simulink model "IndustrialMicrogrid"  (R2023a)
settings: Solver=FixedStepDiscrete  StartTime=0.0  StopTime=10  FixedStep=Ts  RelTol=1e-3
PostLoadFcn:
  | IndustrialMicrogridInputData
  | GfmGridFormingConverterInputParameters
model workspace (MAT data in the model file):
  caseNum = 2
undefined symbols (not defined in the file): base, BESS, DiscIntNeverNeededParam, grid, Grid, gridInverter, machine, microgrid, PV, PVInverter, PVTransformer, scrFactorRg, scrFactorXg, transformer, Ts
libraries: ee_lib x112, eeGeneralControl x104, nesl_utility_internal x64, simulink x56, nesl_utility x37, fl_lib x29, slpidlib x13, eeTransforms x11, eeTotalHarmonicDistorsion x8, eeRmsMeasurement x4, eeSinusoidalMeasurement x4, simulink_extras x2
(part 1 of 14)
CloseFcn:
  | figure1 = findobj('Type', 'figure', 'Name','h1_IndustrialMicrogrid');
  | figure2 = findobj('Type', 'figure', 'Name','h2_IndustrialMicrogrid');
  | figure3 = findobj('Type', 'figure', 'Name','h3_IndustrialMicrogrid');
  | figure4 = findobj('Type', 'figure', 'Name','h4_IndustrialMicrogrid');
  | figure5 = findobj('Type', 'figure', 'Name','h5_IndustrialMicrogrid');
  | close(figure1);
  | close(figure2);
  | close(figure3);
  | close(figure4);
  | close(figure5);
  | clear figure1 figure2 figure3 figure4 figure5
  | clear BESS closedLoop controller currentLoopPole
  | clear fsw_V geometricMean grid Grid inverter KI_PVPLL
  | clear KP_PVPLL logsout_ee_microgrid_resynchronization
  | clear Microgrid PrimaryreactancePV PrimaryresistancePV
  | clear remainingPowerPerString SecondaryreactancePV
  | clear SecondaryresistancePV sensor simlog_ee_microgrid_resynchronization
  | clear simulation solarPanel solarPlant TransformerPrimaryVoltagePV
  | clear TransformerRatingPV TransformerSecondaryVoltagePV
  | clear Ts Ts_V Solar logsout_ee_microgrid_for_mines simlog_ee_microgrid_for_mines
  | clear ans AuxiliaryLoad base BESSCost1 BESSCost2 BESSCost3
  | clear BESSCost4 BESSKVAs1 BESSKVAs2 BESSKVAs3 BESSKVAs4
  | clear BESSMVA1 BESSMVA2 caseNum Conveyor Diesel_cost_s1
  | clear Diesel_cost_s1_yr Diesel_cost_s2 Diesel_cost_s2_yr
  | clear Diesel_cost_s3 Diesel_cost_s3_yr Diesel_cost_s4
  | clear Diesel_cost_s4_yr diesel_litre_USD Diesel_loading_100percent
  | clear Diesel_loading_25percent Diesel_loading_50percent Diesel_loading_75percent
  | clear Diesel_s1 Diesel_s2 Diesel_s3 Diesel_s4 DieselCost1 DieselCost2 DieselCost3
  | clear DieselCost4 DieselKVAs1 DieselKVAs2 DieselKVAs3 DieselKVAs4 DieselMVA
  | clear disturbanceTime DrillingLoad1 DrillingLoad2a DrillingLoad2b Grid1Limited Grid1MVA
  | clear Grid2Limited gridInverter h11a_IndustrialMicrogrid h22a_IndustrialMicrogrid
  | clear h2a_IndustrialMicrogrid imaginaryPart LightingLoad localSolverSampleTime logsout1
  | clear logsout2 logsout3 logsout4 logsout5 logsout_activeloss1 logsout_activeloss2
  | clear logsout_activeloss3 logsout_activeloss4 logsout_activeloss5 logsout_freqmax1
  | clear logsout_freqmax2 logsout_freqmax3 logsout_freqmax4 logsout_freqmax5 logsout_freqmin1
  | clear logsout_freqmin2 logsout_freqmin3 logsout_freqmin4 logsout_freqmin5 logsout_IndustrialMicrogrid
  | clear logsout_LoadTHD1 logsout_LoadTHD2 logsout_LoadTHD3 logsout_LoadTHD4 logsout_LoadTHD5
  | clear logsout_MaxLoadVoltage1 logsout_MaxLoadVoltage2 logsout_MaxLoadVoltage3 logsout_MaxLoadVoltage4
  | clear logsout_MaxLoadVoltage5 logsout_MinLoadVoltage1 logsout_MinLoadVoltage2 logsout_MinLoadVoltage3
  | clear logsout_MinLoadVoltage4 logsout_MinLoadVoltage5 logsout_PCCTHD1 logsout_PCCTHD2
  | clear logsout_PCCTHD3 logsout_PCCTHD4 logsout_PCCTHD5 logsout_reactiveloss1
  | clear logsout_reactiveloss2 logsout_reactiveloss3 logsout_reactiveloss4 logsout_reactiveloss5
  | clear logsout_volmax1 logsout_volmax2 logsout_volmax3 logsout_volmax4 logsout_volmax5
  | clear logsout_volmin1 logsout_volmin2 logsout_volmin3 logsout_volmin4 logsout_volmin5
  | clear machine Machine Micorgrid microgrid op opCase5 ProcessingMotorLoad PV PVCost1
  | clear PVCost2 PVCost3 PVCost4 PVInverter PVKVAs1 PVKVAs2 PVKVAs3 PVKVAs4 PVMVA
  | clear PVTransformer realPart scrFactorRg scrFactorXg scrOut shortCircuit
  | clear simlog_IndustrialMicrogrid simulationTime Solar_cell systemSCR T_on testCondition
  | clear TotalCost1 TotalCost2 TotalCost3 TotalCost4 TotalMG1Load TotalMG2Generation
  | clear TotalMG2Load transformer TransmissionLine tStart tStop voltageLimit voltageLimitMax
  | clear voltageLimitMin XbyROut XbyRtempFactor xlim xticks
  | clear grid Grid gridInverter machine microgrid Microgrid microgridSubsystems PV PVTransformer resultsSubsystems signalRoomSubsystems Ts topLevelSubsystems transformer opCtrlRoomSubsystems
  | clear opCase1 opCase2 opCase3 opCase4 opCase5
Description:
  | Industrial  Microgrid
settings Model: PauseTimes=1  Creator=The MathWorks, Inc.  LastModifiedBy=greed
settings SolverCC: AlgebraicLoopSolver=TrustRegion
settings DataIOCC: ExternalInput=getinputstruct(op)  InitialState=getstatestruct(op)  LoadExternalInput=on  LoadInitialState=on  SaveOutput=off  SaveTime=off  SignalLoggingName=logsout_IndustrialMicrogrid  OutputTimes=[0:1.1*3*Voc/(1*2000):1.1*3*Voc/1]  ReturnWorkspaceOutputsName=simoutData
settings OptimizationCC: ReuseModelBlockBuffer=off
settings DebuggingCC: UnconnectedInputMsg=warning  UnconnectedOutputMsg=warning  UnconnectedLineMsg=warning  StateNameClashWarn=warning  SubsystemReferenceDiagnosticForUnitTest=warning  ArithmeticOperatorsInVariantConditions=warning
settings HardwareCC: ProdBitPerPointer=32  ProdBitPerSizeT=32  ProdBitPerPtrDiffT=32  ProdWordSize=32  ProdHWDeviceType=Intel->x86-32 (Windows32)
settings ModelReferenceCC: EnableRefExpFcnMdlSchedulingChecks=on  PropagateSignalLabelsOutOfModel=off
settings SFSimCC: CustomCodeUndefinedFunction=UseInterfaceOnly
settings RTWCC: DLArmComputeVersion=19.05
settings CodeAppCC: StateflowObjectComments=on
settings SimscapeCC: SimscapeNominalValues="[{\"value\":\"1\",\"unit\":\"A\"},{\"value\":\"1\",\"unit\":\"bar\"},{\"value\":\"1\",\"unit\":\"cm^2\"},{\"value\":\"1\",\"unit\":\"cm^3/s\"},{\"value\":\"1\",\"unit\":\"kJ/kg\"},{\"value\":\"1\",\"unit\":\"kW\"},{\"value\":\"1\",\"unit\":\"l\"},{\"value\":\"1\",\"unit\":\"N\"},{\"value\":\"1\",\"unit\":\"N*m\"},{\"value\":\"1e3\",\"unit\":\"V\"}]"  SimscapeLogType=all  SimscapeLogSimulationStatistics=on  SimscapeLogName=simlog_IndustrialMicrogrid  SimscapeLogLimitData=off

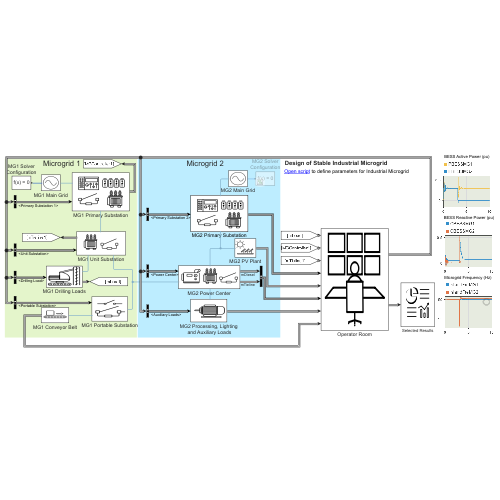
[thumbnail: Simulink's stored preview of the top-level diagram]
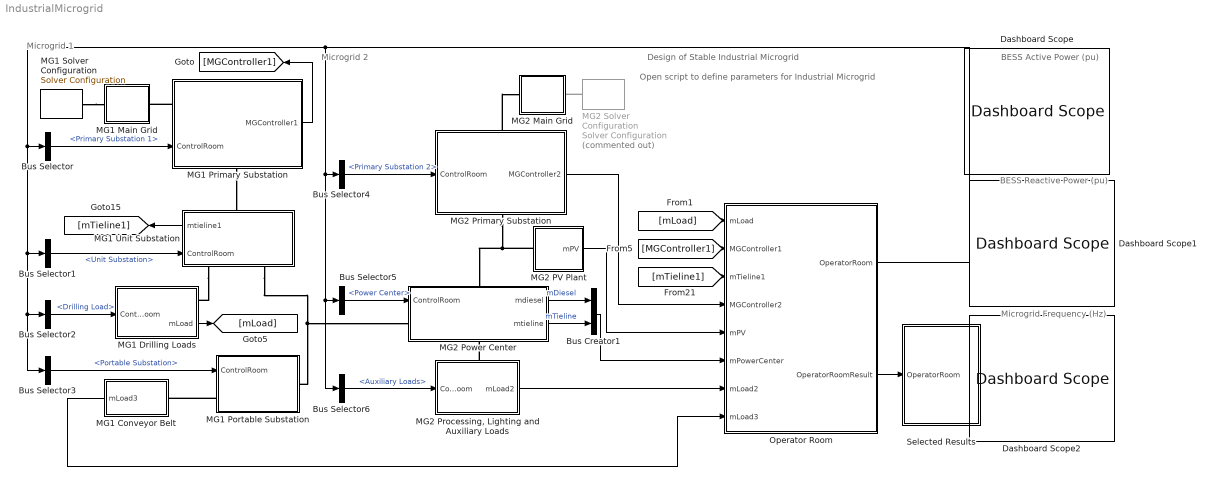
== system IndustrialMicrogrid ==
  note: BESS Active Power (pu)
  note: Microgrid 1
  note: Microgrid 2
  note: Design of Stable Industrial Microgrid
  note: Open script to define parameters for Industrial Microgrid
  note: BESS Reactive Power (pu)
  note: Microgrid Frequency (Hz)
  Bus Creator1 : BusCreator  Inputs=2
  Bus Selector : BusSelector  OutputSignals=Primary Substation 1
  Bus Selector1 : BusSelector  OutputSignals=Unit Substation
  Bus Selector2 : BusSelector  OutputSignals=Drilling Load
  Bus Selector3 : BusSelector  OutputSignals=Portable Substation
  Bus Selector4 : BusSelector  OutputSignals=Primary Substation 2
  Bus Selector5 : BusSelector  OutputSignals=Power Center
  Bus Selector6 : BusSelector  OutputSignals=Auxiliary Loads
  Dashboard Scope : DashboardScope
  Dashboard Scope1 : DashboardScope
  Dashboard Scope2 : DashboardScope
  MG1 Conveyor Belt : Subsystem
      mask Display: image('$imagefile'); % Use "Edit Image" on toolstrip to change.
  MG1 Drilling Loads : Subsystem
      settings: PortSchema="{\"entries\":[{\"content\":{\"sides\":[{\"content\":{\"connectorIds\":[\"In1\"]},\"type\":\"ConnectorPlacement.EquallySpacedRectSide\",\"uuid\":\"8bde343d-193d-4d8c-8111-593ba83965eb\"},{\"content\":{\"connectorIds\":[\"RConn1\",\"Out1\"],\"side\":\"RIGHT\"},\"type\":\"ConnectorPlacement.EquallySpacedRectSide\",\"uuid\":\"2ced8eac-92b1-40fd-b9a3-0c7198a29bec\"},{\"content\":{\"connectorIds\":[],\"side\":\"TOP\"},\"type\":\"ConnectorPlacement.EquallySpacedRectSide\",\"uuid\":\"35b22a7d-ddf4-481a-bb03-3d287fb8e47a\"}]},\"type\":\"ConnectorPlacement.EquallySpacedConnector\",\"uuid\":\"38972ecb-e14c-4d7a-b334-c84224067a82\"}],\"packageUris\":[\"http://schema.mathworks.com/mf0/Connector/R2020b\"],\"version\":\"1.0\"}"
      mask Display: image('$imagefile'); % Use "Edit Image" on toolstrip to change.
  MG1 Main Grid : Subsystem
      mask Display: image('$imagefile'); % Use "Edit Image" on toolstrip to change.
  MG1 Portable Substation : Subsystem
      mask Display: image('$imagefile'); % Use "Edit Image" on toolstrip to change.
  MG1 Primary Substation : Subsystem
      settings: PortSchema="{\"entries\":[{\"content\":{\"sides\":[{\"content\":{\"connectorIds\":[\"LConn1\",\"In1\"]},\"type\":\"ConnectorPlacement.EquallySpacedRectSide\",\"uuid\":\"62c365b4-4668-43f4-b939-0cfa584e512e\"},{\"content\":{\"connectorIds\":[\"Out1\"],\"side\":\"RIGHT\"},\"type\":\"ConnectorPlacement.EquallySpacedRectSide\",\"uuid\":\"025ab869-e565-436b-82b8-3d49f2a71b4a\"},{\"content\":{\"side\":\"TOP\"},\"type\":\"ConnectorPlacement.EquallySpacedRectSide\",\"uuid\":\"be91cdb0-9ff1-46ba-9800-55b3072c8f0d\"},{\"content\":{\"connectorIds\":[\"RConn1\"],\"side\":\"BOTTOM\"},\"type\":\"ConnectorPlacement.EquallySpacedRectSide\",\"uuid\":\"d77b7477-2bba-487e-be1b-8a281c49c410\"}]},\"type\":\"ConnectorPlacement.EquallySpacedConnector\",\"uuid\":\"adc0c184-ac84-487f-a22d-12a7e7737206\"}],\"packageUris\":[\"http://schema.mathworks.com/mf0/Connector/R2020b\"],\"version\":\"1.0\"}"
      mask Display: image('$imagefile'); % Use "Edit Image" on toolstrip to change.
  MG1 Solver Configuration : nesl_utility_internal/Solver Configuration  PhysicalDomain=network_engine_domain  SubClassName=solver  LeftPortType=input  RightPortType=generic  Tones=[]  Harmonics=[]  SimulateNoise=off  Profile=off  UseLocalSampling=off  EnableSwitchedLinearOptims=on  FrequencyDomain=off  UseCCode=off  RelTol=0.001  AbsTol=1e-06  MinStep=1e-09  ToWorkspace=off  RevertToSquareIcSolve=off  NumHomotopyIterations=100  PhasorMode=off  PhasorModeNumHarmonics=1  ConsistencySolver=NEWTON_FTOL  IndexReductionMethod=None  DoDC=off  ResidualTolerance=1e-07  ConsistencyTolSource=GLOBAL  ConsistencyAbsTol=0.001  ConsistencyRelTol=0.001  ConsistencyTolFactor=0.001  UseLocalSolver=on  LocalSolverChoice=NE_PARTITIONING_ADVANCER  ResolveIndetEquations=on  FunctionEvalNumThread=1  LocalSolverSampleTime=Ts  DoFixedCost=on  MaxNonlinIter=3  MaxModeIter=2  ComputeImpulses=off  ImpulseIterations=1  LinearAlgebra=auto  LinearAlgebraNumThread=0  EquationFormulation=NE_TIME_EF  DelaysMemoryBudget=1024  AutomaticFiltering=off  FilteringTimeConstant=0.001  PartitionStorageMethod=EXHAUSTIVE  PartitionMemoryBudget=1024  PartitionMethod=ROBUST
  MG1 Unit Substation : Subsystem
      settings: PortSchema="{\"entries\":[{\"content\":{\"sides\":[{\"content\":{\"connectorIds\":[\"Out1\",\"In1\"]},\"type\":\"ConnectorPlacement.EquallySpacedRectSide\",\"uuid\":\"75ac93d6-cc6a-445c-be45-fffab924bfd7\"},{\"content\":{\"side\":\"RIGHT\"},\"type\":\"ConnectorPlacement.EquallySpacedRectSide\",\"uuid\":\"e5c53324-ad77-49da-90c4-df6ba5240965\"},{\"content\":{\"connectorIds\":[\"LConn1\"],\"side\":\"TOP\"},\"type\":\"ConnectorPlacement.EquallySpacedRectSide\",\"uuid\":\"55d13e88-751b-43c7-af74-511b72769f16\"},{\"content\":{\"connectorIds\":[\"RConn1\",\"RConn2\"],\"side\":\"BOTTOM\"},\"type\":\"ConnectorPlacement.EquallySpacedRectSide\",\"uuid\":\"b5dd3cb9-7b98-4c05-8dd8-d8e7dc6e0ca9\"}]},\"type\":\"ConnectorPlacement.EquallySpacedConnector\",\"uuid\":\"f5372cf6-2eab-4920-89a5-bce690804323\"}],\"packageUris\":[\"http://schema.mathworks.com/mf0/Connector/R2020b\"],\"version\":\"1.0\"}"
      mask Display: image('$imagefile'); % Use "Edit Image" on toolstrip to change.
  MG2 Main Grid : Subsystem
      mask Display: image('$imagefile'); % Use "Edit Image" on toolstrip to change.
  MG2 PV Plant : Subsystem
      mask Display: image('$imagefile'); % Use "Edit Image" on toolstrip to change.
  MG2 Power Center : Subsystem
      settings: PortSchema="{\"entries\":[{\"content\":{\"sides\":[{\"content\":{\"connectorIds\":[\"In1\",\"LConn1\"]},\"type\":\"ConnectorPlacement.EquallySpacedRectSide\",\"uuid\":\"75ac93d6-cc6a-445c-be45-fffab924bfd7\"},{\"content\":{\"connectorIds\":[\"Out1\",\"Out2\"],\"side\":\"RIGHT\"},\"type\":\"ConnectorPlacement.EquallySpacedRectSide\",\"uuid\":\"e5c53324-ad77-49da-90c4-df6ba5240965\"},{\"content\":{\"connectorIds\":[\"LConn2\"],\"side\":\"TOP\"},\"type\":\"ConnectorPlacement.EquallySpacedRectSide\",\"uuid\":\"55d13e88-751b-43c7-af74-511b72769f16\"},{\"content\":{\"connectorIds\":[\"RConn1\"],\"side\":\"BOTTOM\"},\"type\":\"ConnectorPlacement.EquallySpacedRectSide\",\"uuid\":\"640896eb-fba6-44de-a484-c435c51ba156\"}]},\"type\":\"ConnectorPlacement.EquallySpacedConnector\",\"uuid\":\"f5372cf6-2eab-4920-89a5-bce690804323\"}],\"packageUris\":[\"http://schema.mathworks.com/mf0/Connector/R2020b\"],\"version\":\"1.0\"}"
      mask Display: image('$imagefile'); % Use "Edit Image" on toolstrip to change.
  MG2 Primary Substation : Subsystem
      settings: PortSchema="{\"entries\":[{\"content\":{\"sides\":[{\"content\":{\"connectorIds\":[\"In1\"]},\"type\":\"ConnectorPlacement.EquallySpacedRectSide\",\"uuid\":\"a418e4cb-bf63-409d-8e7f-8f8f381466aa\"},{\"content\":{\"connectorIds\":[\"Out1\"],\"side\":\"RIGHT\"},\"type\":\"ConnectorPlacement.EquallySpacedRectSide\",\"uuid\":\"36367aff-fc5a-4e64-9409-cab392a29391\"},{\"content\":{\"connectorIds\":[\"LConn1\"],\"side\":\"TOP\"},\"type\":\"ConnectorPlacement.EquallySpacedRectSide\",\"uuid\":\"594bd116-4459-44f1-a349-157ea2209965\"},{\"content\":{\"connectorIds\":[\"RConn1\"],\"side\":\"BOTTOM\"},\"type\":\"ConnectorPlacement.EquallySpacedRectSide\",\"uuid\":\"1ed5e2c8-52ef-46e8-a3fd-2e92dd02a56f\"}]},\"type\":\"ConnectorPlacement.EquallySpacedConnector\",\"uuid\":\"f6551318-b622-4306-bcf5-d56dd1a3ddaf\"}],\"packageUris\":[\"http://schema.mathworks.com/mf0/Connector/R2020b\"],\"version\":\"1.0\"}"
      mask Display: image('$imagefile'); % Use "Edit Image" on toolstrip to change.
  "MG2 Processing, Lighting and Auxiliary Loads" : Subsystem
      settings: PortSchema="{\"entries\":[{\"content\":{\"sides\":[{\"content\":{\"connectorIds\":[\"In1\"]},\"type\":\"ConnectorPlacement.EquallySpacedRectSide\",\"uuid\":\"8bde343d-193d-4d8c-8111-593ba83965eb\"},{\"content\":{\"connectorIds\":[\"Out1\"],\"side\":\"RIGHT\"},\"type\":\"ConnectorPlacement.EquallySpacedRectSide\",\"uuid\":\"2ced8eac-92b1-40fd-b9a3-0c7198a29bec\"},{\"content\":{\"connectorIds\":[\"LConn1\"],\"side\":\"TOP\"},\"type\":\"ConnectorPlacement.EquallySpacedRectSide\",\"uuid\":\"35b22a7d-ddf4-481a-bb03-3d287fb8e47a\"}]},\"type\":\"ConnectorPlacement.EquallySpacedConnector\",\"uuid\":\"38972ecb-e14c-4d7a-b334-c84224067a82\"}],\"packageUris\":[\"http://schema.mathworks.com/mf0/Connector/R2020b\"],\"version\":\"1.0\"}"
      mask Display: image('$imagefile'); % Use "Edit Image" on toolstrip to change.
  MG2 Solver Configuration : nesl_utility_internal/Solver Configuration  Commented=on  PhysicalDomain=network_engine_domain  SubClassName=solver  LeftPortType=input  RightPortType=generic  Tones=[]  Harmonics=[]  SimulateNoise=off  Profile=off  UseLocalSampling=off  EnableSwitchedLinearOptims=on  FrequencyDomain=off  UseCCode=off  RelTol=0.001  AbsTol=1e-06  MinStep=1e-09  ToWorkspace=off  RevertToSquareIcSolve=off  NumHomotopyIterations=100  PhasorMode=off  PhasorModeNumHarmonics=1  ConsistencySolver=NEWTON_FTOL  IndexReductionMethod=None  DoDC=off  ResidualTolerance=1e-07  ConsistencyTolSource=GLOBAL  ConsistencyAbsTol=0.001  ConsistencyRelTol=0.001  ConsistencyTolFactor=0.001  UseLocalSolver=on  LocalSolverChoice=NE_PARTITIONING_ADVANCER  ResolveIndetEquations=on  FunctionEvalNumThread=1  LocalSolverSampleTime=Ts  DoFixedCost=on  MaxNonlinIter=3  MaxModeIter=2  ComputeImpulses=off  ImpulseIterations=1  LinearAlgebra=auto  LinearAlgebraNumThread=0  EquationFormulation=NE_TIME_EF  DelaysMemoryBudget=1024  AutomaticFiltering=off  FilteringTimeConstant=0.001  PartitionStorageMethod=EXHAUSTIVE  PartitionMemoryBudget=1024  PartitionMethod=ROBUST
  Operator Room : Subsystem
      mask Display: image('$imagefile'); % Use "Edit Image" on toolstrip to change.
  Selected Results : Subsystem
      mask Display: image('$imagefile'); % Use "Edit Image" on toolstrip to change.
  wires:
  MG1 Primary Substation/1(MGController1) -> [MGController1]
  MG1 Drilling Loads/1(mLoad) -> [mLoad]
  Bus Selector1/1 -> MG1 Unit Substation/1(ControlRoom)  "<Unit Substation>"
  Bus Selector2/1 -> MG1 Drilling Loads/1(ControlRoom)  "<Drilling Load>"
  Bus Selector3/1 -> MG1 Portable Substation/1(ControlRoom)  "<Portable Substation>"
  [mLoad] -> Operator Room/1(mLoad)
  "MG2 Processing, Lighting and Auxiliary Loads"/1(mLoad2) -> Operator Room/7(mLoad2)
  MG2 Primary Substation/1(MGController2) -> Operator Room/4(MGController2)
  MG2 PV Plant/1(mPV) -> Operator Room/5(mPV)
  [MGController1] -> Operator Room/2(MGController1)
  MG1 Conveyor Belt/1(mLoad3) -> Operator Room/8(mLoad3)
  MG1 Unit Substation/1(mtieline1) -> [mTieline1]
  Operator Room/1(OperatorRoom) -> Bus Selector6/1, Bus Selector5/1, Bus Selector4/1, Bus Selector2/1, Bus Selector3/1, Bus Selector1/1, Bus Selector/1
  Bus Selector5/1 -> MG2 Power Center/1(ControlRoom)  "<Power Center>"
  Bus Selector6/1 -> "MG2 Processing, Lighting and Auxiliary Loads"/1(ControlRoom)  "<Auxiliary Loads>"
  Bus Selector/1 -> MG1 Primary Substation/1(ControlRoom)  "<Primary Substation 1>"
  MG2 Power Center/1(mdiesel) -> Bus Creator1/1  "mDiesel"
  MG2 Power Center/2(mtieline) -> Bus Creator1/2  "mTieline"
  Operator Room/2(OperatorRoomResult) -> Selected Results/1(OperatorRoom)
  [mTieline1] -> Operator Room/3(mTieline1)
  Bus Creator1/1 -> Operator Room/6(mPowerCenter)
  Bus Selector4/1 -> MG2 Primary Substation/1(ControlRoom)  "<Primary Substation 2>"
  connections:
  MG1 Primary Substation/LConn1 -- MG1 Main Grid/RConn1
  MG1 Solver Configuration/RConn1 -- MG1 Main Grid/LConn1
  MG1 Primary Substation/RConn1 -- MG1 Unit Substation/LConn1
  MG2 Solver Configuration/RConn1 -- MG2 Main Grid/LConn1
  "MG2 Processing, Lighting and Auxiliary Loads"/LConn1 -- MG2 Power Center/RConn1
  MG2 Primary Substation/LConn1 -- MG2 Main Grid/RConn1
  MG1 Unit Substation/RConn1 -- MG1 Drilling Loads/RConn1
  MG1 Unit Substation/RConn2 -- MG1 Portable Substation/RConn1 -- MG2 Power Center/LConn1
  MG1 Portable Substation/LConn1 -- MG1 Conveyor Belt/LConn1
  MG2 Primary Substation/RConn1 -- MG2 PV Plant/LConn1 -- MG2 Power Center/LConn2

== system IndustrialMicrogrid/MG1 Conveyor Belt ==
  Average-Value Rectifier (Three-Phase) : ee_lib/Semiconductors & Converters/Converters/Average-Value Rectifier (Three-Phase)  port_option=ee.enum.threePhasePort.composite  frequency_option=ee.enum.converters.frequency.variable  VRated=microgrid.powerCenterTransformerSecondaryVoltage V  FRated=60 Hz  Pfixed=5e3 W
      settings: InternalSimscapePortConfiguration="{\"Bottom\":[],\"Left\":[{\"id\":\"N\",\"label\":\"~\",\"type\":\"foundation.electrical.three_phase\"}],\"Right\":[{\"id\":\"p\",\"label\":\"+\",\"type\":\"foundation.electrical.electrical\"},{\"id\":\"n\",\"label\":\"-\",\"type\":\"foundation.electrical.electrical\"}],\"Top\":[]}"
  Low-Pass Filter (Discrete or Continuous)1 : eeGeneralControl/Low-Pass Filter (Discrete or Continuous)  K=1  T=0.02  B=inf  A=-inf  init_option=Inherited from block input  x0=0  Ts=Ts
  Low-Pass Filter (Discrete or Continuous)2 : eeGeneralControl/Low-Pass Filter (Discrete or Continuous)  K=1  T=0.02  B=inf  A=-inf  init_option=Inherited from block input  x0=0  Ts=Ts
  PS-Simulink Converter6 : nesl_utility_internal/PS-Simulink Converter  PhysicalDomain=network_engine_domain  SubClassName=ps_output  LeftPortType=input  RightPortType=output  PseudoPeriodic=off  Frequencies=[]  VectorFormat=1-D array  Unit=MW  AffineConversion=off
  PS-Simulink Converter7 : nesl_utility_internal/PS-Simulink Converter  PhysicalDomain=network_engine_domain  SubClassName=ps_output  LeftPortType=input  RightPortType=output  PseudoPeriodic=off  Frequencies=[]  VectorFormat=1-D array  Unit=MV*A  AffineConversion=off
  Power Sensor (Three-Phase)1 : ee_lib/Sensors & Transducers/Power Sensor (Three-Phase)  load_type=ee.enum.passive.type_balanced.balanced  f0=60 Hz  config=ee.enum.with_neutral.no  rho=1
      settings: InternalSimscapePortConfiguration="{\"Bottom\":[],\"Left\":[{\"id\":\"N1\",\"label\":\"~1\",\"type\":\"foundation.electrical.three_phase\"}],\"Right\":[{\"id\":\"N2\",\"label\":\"~2\",\"type\":\"foundation.electrical.three_phase\"}],\"Top\":[{\"id\":\"Pm\",\"label\":\"P\",\"type\":\"output\"},{\"id\":\"Qm\",\"label\":\"Q\",\"type\":\"output\"}]}"
  Resistor : ee_lib/Passive/Resistor  R=2500 Ohm  enable_R_tol=0  R_tol=5  tol_distribution=1  nSigma=4  enable_operating_limits=0  operating_limit_action=2  power_rating=1 W  max_working_voltage=100 V  enable_faults=ee.enum.enable.no  fault_action=simscape.enum.assert.action.none  R_faulted=inf Ohm  fault_trigger=ee.enum.faults.faultTrigger.temporal  t_fault=1 s  max_permissible_current=1 A  t_fail_on_current=1 s  noise_mode=0  Tdevice=25 degC  sample_time=1e-3 s  repeatability=1  user_seed=0  auto_seed=3499211588  power_derating_T1=70 degC  power_derating_T2=155 degC  operating_temperature_range_vec=[-50, 150] degC  alpha=3.93e-3 1/K  Tmeas=25 degC  thermal_mass=100 J/K  temperature_specify=off  temperature_priority=High  temperature=298.15 K  temperature_nominal_specify=off  temperature_nominal_unit=K  temperature_nominal_value=1
  ~ : PMIOPort  Side=Left
  Out Bus Element2 : Outport  PortName=mLoad3  Element=activepower
  Out Bus Element3 : Outport  PortName=mLoad3  Element=reactivepower
  wires:
  PS-Simulink Converter6/1 -> Low-Pass Filter (Discrete or Continuous)1/1
  PS-Simulink Converter7/1 -> Low-Pass Filter (Discrete or Continuous)2/1
  Low-Pass Filter (Discrete or Continuous)1/1 -> Out Bus Element2/1
  Low-Pass Filter (Discrete or Continuous)2/1 -> Out Bus Element3/1
  connections:
  Resistor/LConn1 -- Average-Value Rectifier (Three-Phase)/RConn1
  Resistor/RConn1 -- Average-Value Rectifier (Three-Phase)/RConn2
  ~/RConn1 -- Power Sensor (Three-Phase)1/LConn1
  Power Sensor (Three-Phase)1/RConn1 -- Average-Value Rectifier (Three-Phase)/LConn1
  Power Sensor (Three-Phase)1/LConn2 -- PS-Simulink Converter6/LConn1
  Power Sensor (Three-Phase)1/LConn3 -- PS-Simulink Converter7/LConn1

== system IndustrialMicrogrid/MG1 Drilling Loads ==
  Bus Element In3 : Inport  PortName=ControlRoom  Element=Load2aControl
  Bus Element In1 : Inport  PortName=ControlRoom  Element=Load1Control
  Bus Element In2 : Inport  PortName=ControlRoom  Element=Load2bControl
  Circuit Breaker (Three-Phase)1 : ee_lib/Switches & Breakers/Circuit Breaker (Three-Phase)  R_closed=0.001 Ohm  G_open=1e-6 1/Ohm  threshold=0.5 V  breaker_behavior=ee.enum.switches.breakerBehavior.zeroCrossingEnable
      settings: InternalSimscapePortConfiguration="{\"Bottom\":[],\"Left\":[{\"id\":\"vT\",\"label\":\"vT\",\"type\":\"input\"},{\"id\":\"N1\",\"label\":\"~1\",\"type\":\"foundation.electrical.three_phase\"}],\"Right\":[{\"id\":\"N2\",\"label\":\"~2\",\"type\":\"foundation.electrical.three_phase\"}],\"Top\":[]}"
  Circuit Breaker (Three-Phase)2 : ee_lib/Switches & Breakers/Circuit Breaker (Three-Phase)  R_closed=0.001 Ohm  G_open=1e-6 1/Ohm  threshold=0.5 V  breaker_behavior=ee.enum.switches.breakerBehavior.zeroCrossingEnable
      settings: InternalSimscapePortConfiguration="{\"Bottom\":[],\"Left\":[{\"id\":\"vT\",\"label\":\"vT\",\"type\":\"input\"},{\"id\":\"N1\",\"label\":\"~1\",\"type\":\"foundation.electrical.three_phase\"}],\"Right\":[{\"id\":\"N2\",\"label\":\"~2\",\"type\":\"foundation.electrical.three_phase\"}],\"Top\":[]}"
  Circuit Breaker (Three-Phase)3 : ee_lib/Switches & Breakers/Circuit Breaker (Three-Phase)  R_closed=0.001 Ohm  G_open=1e-6 1/Ohm  threshold=0.5 V  breaker_behavior=ee.enum.switches.breakerBehavior.zeroCrossingEnable
      settings: InternalSimscapePortConfiguration="{\"Bottom\":[],\"Left\":[{\"id\":\"vT\",\"label\":\"vT\",\"type\":\"input\"},{\"id\":\"N1\",\"label\":\"~1\",\"type\":\"foundation.electrical.three_phase\"}],\"Right\":[{\"id\":\"N2\",\"label\":\"~2\",\"type\":\"foundation.electrical.three_phase\"}],\"Top\":[]}"
  Electrical Reference1 : fl_lib/Electrical/Electrical Elements/Electrical Reference
  Electrical Reference2 : fl_lib/Electrical/Electrical Elements/Electrical Reference
  Load Measurements1 : Subsystem
  Simulink-PS Converter1 : nesl_utility_internal/Simulink-PS Converter  PhysicalDomain=network_engine_domain  SubClassName=ps_input  LeftPortType=input  RightPortType=output  PseudoPeriodic=off  Frequencies=[]  NoiseDistribution=none  NoiseParameters=[]  Unit=1  AffineConversion=off  FilteringAndDerivatives=provide  SimscapeFilterOrder=1  InputFilterTimeConstant=0.001  UdotUserProvided=0
  Simulink-PS Converter2 : nesl_utility_internal/Simulink-PS Converter  PhysicalDomain=network_engine_domain  SubClassName=ps_input  LeftPortType=input  RightPortType=output  PseudoPeriodic=off  Frequencies=[]  NoiseDistribution=none  NoiseParameters=[]  Unit=1  AffineConversion=off  FilteringAndDerivatives=provide  SimscapeFilterOrder=1  InputFilterTimeConstant=0.001  UdotUserProvided=0
  Simulink-PS Converter3 : nesl_utility_internal/Simulink-PS Converter  PhysicalDomain=network_engine_domain  SubClassName=ps_input  LeftPortType=input  RightPortType=output  PseudoPeriodic=off  Frequencies=[]  NoiseDistribution=none  NoiseParameters=[]  Unit=1  AffineConversion=off  FilteringAndDerivatives=provide  SimscapeFilterOrder=1  InputFilterTimeConstant=0.001  UdotUserProvided=0
  Subsystem2 : Subsystem
  Switchable 105 kW 460 Vrms 60 Hz : ee_lib/Passive/RLC Assemblies/Wye-Connected Load  parameterization=ee.enum.rlc.parameterization.ratedpower  component_structure=ee.enum.rlc.structure.C  component_structure_PQ=ee.enum.rlc.structure.SeriesRL  R=1 Ohm  L=0.001 H  C=1e-6 F  VRated=microgrid.unitSubstationVoltage V  FRated=microgrid.frequency Hz  P=microgrid.pLoad1*0.25 W  Qpos=microgrid.qLoad1*0.5 A*V  Qneg=-3000 A*V  R_parasitic=1e-6 Ohm  G_parasitic=1e-6 1/Ohm  R_parasitic_PQ=1e-6 Ohm  G_parasitic_PQ=1e-6 1/Ohm  Vmag0=0 V  Vang0=0 deg  Freq0=microgrid.frequency Hz  IL_specify=on  IL_priority=High  IL=[ 0 0 0 ] A  IL_nominal_specify=off  IL_nominal_unit=A  IL_nominal_value=1  VC_specify=on  VC_priority=High  VC=[ 0 0 0 ] V  VC_nominal_specify=off  VC_nominal_unit=V  VC_nominal_value=1
  Switchable 105 kW 460 Vrms 60 Hz1 : ee_lib/Passive/RLC Assemblies/Wye-Connected Load  parameterization=ee.enum.rlc.parameterization.ratedpower  component_structure=ee.enum.rlc.structure.C  component_structure_PQ=ee.enum.rlc.structure.SeriesRL  R=1 Ohm  L=0.001 H  C=1e-6 F  VRated=microgrid.unitSubstationVoltage V  FRated=microgrid.frequency Hz  P=microgrid.pLoad1*0.25 W  Qpos=microgrid.qLoad1*0.5 A*V  Qneg=-3000 A*V  R_parasitic=1e-6 Ohm  G_parasitic=1e-6 1/Ohm  R_parasitic_PQ=1e-6 Ohm  G_parasitic_PQ=1e-6 1/Ohm  Vmag0=0 V  Vang0=0 deg  Freq0=microgrid.frequency Hz  IL_specify=on  IL_priority=High  IL=[ 0 0 0 ] A  IL_nominal_specify=off  IL_nominal_unit=A  IL_nominal_value=1  VC_specify=on  VC_priority=High  VC=[ 0 0 0 ] V  VC_nominal_specify=off  VC_nominal_unit=V  VC_nominal_value=1
  ~ : PMIOPort  Side=Right
  mLoad : Outport
  wires:
  Bus Element In3/1 -> Simulink-PS Converter1/1
  Bus Element In1/1 -> Simulink-PS Converter3/1
  Load Measurements1/1(mLoad) -> mLoad/1
  Bus Element In2/1 -> Simulink-PS Converter2/1
  connections:
  Circuit Breaker (Three-Phase)1/RConn1 -- Switchable 105 kW 460 Vrms 60 Hz/LConn1
  ~/RConn1 -- Load Measurements1/LConn1
  Simulink-PS Converter1/RConn1 -- Circuit Breaker (Three-Phase)2/LConn1
  Circuit Breaker (Three-Phase)1/LConn2 -- Circuit Breaker (Three-Phase)3/LConn2 -- Circuit Breaker (Three-Phase)2/LConn2 -- Load Measurements1/RConn1
  Simulink-PS Converter3/RConn1 -- Circuit Breaker (Three-Phase)1/LConn1
  Electrical Reference2/LConn1 -- Switchable 105 kW 460 Vrms 60 Hz/RConn1
  Circuit Breaker (Three-Phase)2/RConn1 -- Switchable 105 kW 460 Vrms 60 Hz1/LConn1
  Simulink-PS Converter2/RConn1 -- Circuit Breaker (Three-Phase)3/LConn1
  Switchable 105 kW 460 Vrms 60 Hz1/RConn1 -- Electrical Reference1/LConn1
  Circuit Breaker (Three-Phase)3/RConn1 -- Subsystem2/RConn1

== system IndustrialMicrogrid/MG1 Main Grid ==
  Delta-Connected Load : ee_lib/Passive/RLC Assemblies/Delta-Connected Load  parameterization=ee.enum.rlc.parameterization.ratedpower  component_structure=ee.enum.rlc.structure.R  component_structure_PQ=ee.enum.rlc.structure.SeriesRL  R=1 Ohm  L=1e-3 H  C=1e-6 F  VRated=grid.voltage V  FRated=grid.frequency Hz  P=grid.pLoad kW  Qpos=grid.qLoad A*V  Qneg=-1e2 A*V  R_parasitic=1e-6 Ohm  G_parasitic=1e-6 1/Ohm  R_parasitic_PQ=1e-6 Ohm  G_parasitic_PQ=1e-6 1/Ohm  Vmag0=grid.voltage V  Vang0=0 deg  Freq0=grid.frequency Hz  IL_specify=off  IL_priority=High  IL=[0, 0, 0] A  IL_nominal_specify=off  IL_nominal_unit=A  IL_nominal_value=1  VC_specify=off  VC_priority=High  VC=[0, 0, 0] V  VC_nominal_specify=off  VC_nominal_unit=V  VC_nominal_value=1
      settings: InternalSimscapePortConfiguration="{\"Bottom\":[],\"Left\":[{\"id\":\"N\",\"label\":\"~\",\"type\":\"foundation.electrical.three_phase\"}],\"Right\":[],\"Top\":[]}"
  Electrical Reference3 : fl_lib/Electrical/Electrical Elements/Electrical Reference
  Main Grid Frequency : Constant  Value=grid.frequency  SampleTime=-1
  Programmable Voltage Source (Three-Phase)2 : ee_lib/Sources/Programmable Voltage Source (Three-Phase)  magnitude_type=ee.enum.timechanging.constant  vline_rms=grid.voltageSource V  magn_ramp=1 V/s  magn_step=1 V  magn_modu_magn=1 V  magn_modu_freq=1 Hz  magn_t1=1 s  magn_t2=2 s  frequency_type=ee.enum.timechanging.external  freq=50 Hz  freq_ramp=1 Hz/s  freq_step=1 Hz  freq_modu_magn=1 Hz  freq_modu_freq=1 Hz  freq_t1=1 s  freq_t2=2 s  phase_type=ee.enum.timechanging.constant  shift=0 deg  phase_ramp=1 deg/s  phase_step=1 deg  phase_modu_magn=1 deg  phase_modu_freq=1 Hz  phase_t1=1 s  phase_t2=2 s  impedance_option=1  SShortCircuit=100e6 A*V  XR=15  R=Grid.Resistance Ohm  L=3.97e-4 H  G_parasitic=1e-6 1/Ohm  harmonic_option=0  harmonic_orders=[5, 7, 11, 13]  harmonic_ratios=[.1, .1, .1, .1]  harmonic_shifts=[0, 0, 0, 0] deg  harmonic_sequences=[1, 1, 1, 1]  harmonic_t1=-inf s  harmonic_t2=inf s  I_specify=on  I_priority=None  I=[0, 0, 0] A  I_nominal_specify=off  I_nominal_unit=A  I_nominal_value=1  V_specify=on  V_priority=None  V=[0, 0, 0] V  V_nominal_specify=off  V_nominal_unit=V  V_nominal_value=1
      settings: InternalSimscapePortConfiguration="{\"Bottom\":[],\"Left\":[{\"id\":\"ext_freq\",\"label\":\"F\",\"type\":\"input\"},{\"id\":\"n\",\"label\":\"n\",\"type\":\"foundation.electrical.electrical\"}],\"Right\":[{\"id\":\"N\",\"label\":\"~\",\"type\":\"foundation.electrical.three_phase\"}],\"Top\":[]}"
  Simulink-PS Converter : nesl_utility_internal/Simulink-PS Converter  PhysicalDomain=network_engine_domain  SubClassName=ps_input  LeftPortType=input  RightPortType=output  PseudoPeriodic=off  Frequencies=[]  NoiseDistribution=none  NoiseParameters=[]  Unit=1  AffineConversion=off  FilteringAndDerivatives=provide  SimscapeFilterOrder=1  InputFilterTimeConstant=0.001  UdotUserProvided=0
  Source impedance and Line X/R=18.8 : ee_lib/Passive/RLC Assemblies/RLC (Three-Phase)  component_structure=ee.enum.rlc.structure.SeriesRL  R=grid.rMV Ohm  L=grid.lMV H  C=1e-6 F  R_parasitic=1e-6 Ohm  G_parasitic=1e-6 1/Ohm  IL_specify=on  IL_priority=High  IL=[0, 0, 0] A  IL_nominal_specify=off  IL_nominal_unit=A  IL_nominal_value=1  VC_specify=off  VC_priority=High  VC=[0, 0, 0] V  VC_nominal_specify=off  VC_nominal_unit=V  VC_nominal_value=1
      settings: InternalSimscapePortConfiguration="{\"Bottom\":[],\"Left\":[{\"id\":\"N1\",\"label\":\"~1\",\"type\":\"foundation.electrical.three_phase\"}],\"Right\":[{\"id\":\"N2\",\"label\":\"~2\",\"type\":\"foundation.electrical.three_phase\"}],\"Top\":[]}"
  ref : PMIOPort  Side=Left
  ~ : PMIOPort  Port=2  Side=Right
  wires:
  Main Grid Frequency/1 -> Simulink-PS Converter/1
  connections:
  Simulink-PS Converter/RConn1 -- Programmable Voltage Source (Three-Phase)2/LConn1
  Delta-Connected Load/LConn1 -- ~/RConn1 -- Source impedance and Line X/R=18.8/RConn1
  Source impedance and Line X/R=18.8/LConn1 -- Programmable Voltage Source (Three-Phase)2/RConn1
  ref/RConn1 -- Electrical Reference3/LConn1 -- Programmable Voltage Source (Three-Phase)2/LConn2

== system IndustrialMicrogrid/MG1 Portable Substation ==
  Bus Element In3 : Inport  PortName=ControlRoom  Element=PortableSubstationBrk1
  Circuit Breaker (Three-Phase)1 : ee_lib/Switches & Breakers/Circuit Breaker (Three-Phase)  R_closed=0.001 Ohm  G_open=1e-6 1/Ohm  threshold=0.5 V  breaker_behavior=ee.enum.switches.breakerBehavior.zeroCrossingEnable
      settings: InternalSimscapePortConfiguration="{\"Bottom\":[],\"Left\":[{\"id\":\"vT\",\"label\":\"vT\",\"type\":\"input\"},{\"id\":\"N1\",\"label\":\"~1\",\"type\":\"foundation.electrical.three_phase\"}],\"Right\":[{\"id\":\"N2\",\"label\":\"~2\",\"type\":\"foundation.electrical.three_phase\"}],\"Top\":[]}"
  Line X/R=1.44 1 : ee_lib/Passive/RLC Assemblies/RLC (Three-Phase)  component_structure=ee.enum.rlc.structure.SeriesRL  R=microgrid.rLine*1.2 Ohm  L=microgrid.lLine*1.2 H  C=1 F  R_parasitic=1e-6 Ohm  G_parasitic=1e-5 1/Ohm  IL_specify=on  IL_priority=High  IL=[0, 0, 0] A  IL_nominal_specify=off  IL_nominal_unit=A  IL_nominal_value=1  VC_specify=on  VC_priority=High  VC=[0, 0, 0] V  VC_nominal_specify=off  VC_nominal_unit=V  VC_nominal_value=1
      settings: InternalSimscapePortConfiguration="{\"Bottom\":[],\"Left\":[{\"id\":\"N1\",\"label\":\"~1\",\"type\":\"foundation.electrical.three_phase\"}],\"Right\":[{\"id\":\"N2\",\"label\":\"~2\",\"type\":\"foundation.electrical.three_phase\"}],\"Top\":[]}"
  Line X/R=1.44 2 : ee_lib/Passive/RLC Assemblies/RLC (Three-Phase)  component_structure=ee.enum.rlc.structure.SeriesRL  R=microgrid.rLine*0.2 Ohm  L=microgrid.lLine*0.2 H  C=1 F  R_parasitic=1e-6 Ohm  G_parasitic=1e-5 1/Ohm  IL_specify=on  IL_priority=High  IL=[0, 0, 0] A  IL_nominal_specify=off  IL_nominal_unit=A  IL_nominal_value=1  VC_specify=on  VC_priority=High  VC=[0, 0, 0] V  VC_nominal_specify=off  VC_nominal_unit=V  VC_nominal_value=1
      settings: InternalSimscapePortConfiguration="{\"Bottom\":[],\"Left\":[{\"id\":\"N1\",\"label\":\"~1\",\"type\":\"foundation.electrical.three_phase\"}],\"Right\":[{\"id\":\"N2\",\"label\":\"~2\",\"type\":\"foundation.electrical.three_phase\"}],\"Top\":[]}"
  Simulink-PS Converter : nesl_utility_internal/Simulink-PS Converter  PhysicalDomain=network_engine_domain  SubClassName=ps_input  LeftPortType=input  RightPortType=output  PseudoPeriodic=off  Frequencies=[]  NoiseDistribution=none  NoiseParameters=[]  Unit=1  AffineConversion=off  FilteringAndDerivatives=provide  SimscapeFilterOrder=1  InputFilterTimeConstant=0.001  UdotUserProvided=0
  "~ " : PMIOPort  Side=Left
  Conn1 : PMIOPort  Port=2  Side=Right
  wires:
  Bus Element In3/1 -> Simulink-PS Converter/1
  connections:
  Line X/R=1.44 2/LConn1 -- "~ "/RConn1
  Circuit Breaker (Three-Phase)1/RConn1 -- Line X/R=1.44 1/LConn1
  Circuit Breaker (Three-Phase)1/LConn1 -- Simulink-PS Converter/RConn1
  Circuit Breaker (Three-Phase)1/LConn2 -- Line X/R=1.44 2/RConn1
  Line X/R=1.44 1/RConn1 -- Conn1/RConn1

== system IndustrialMicrogrid/MG1 Primary Substation ==
  ControlRoom : Inport
  BESS and Controller : Subsystem
  Bus Creator : BusCreator  Inputs=2
  Bus Selector : BusSelector  OutputSignals=SubstationBrk
  Circuit Breaker (Three-Phase) : ee_lib/Switches & Breakers/Circuit Breaker (Three-Phase)  R_closed=0.001 Ohm  G_open=1e-6 1/Ohm  threshold=0.5 V  breaker_behavior=ee.enum.switches.breakerBehavior.zeroCrossingEnable
      settings: InternalSimscapePortConfiguration="{\"Bottom\":[],\"Left\":[{\"id\":\"vT\",\"label\":\"vT\",\"type\":\"input\"},{\"id\":\"N1\",\"label\":\"~1\",\"type\":\"foundation.electrical.three_phase\"}],\"Right\":[{\"id\":\"N2\",\"label\":\"~2\",\"type\":\"foundation.electrical.three_phase\"}],\"Top\":[]}"
  Microgrid Controller : Subsystem
  PCC Measurements and PCC Breaker : Subsystem
      mask Display: image('$imagefile'); % Use "Edit Image" on toolstrip to change.
  Simulink-PS Converter : nesl_utility_internal/Simulink-PS Converter  PhysicalDomain=network_engine_domain  SubClassName=ps_input  LeftPortType=input  RightPortType=output  PseudoPeriodic=off  Frequencies=[]  NoiseDistribution=none  NoiseParameters=[]  Unit=1  AffineConversion=off  FilteringAndDerivatives=provide  SimscapeFilterOrder=1  InputFilterTimeConstant=0.001  UdotUserProvided=0
  Transformer and Disconnectors : Subsystem
      mask Display: image('$imagefile'); % Use "Edit Image" on toolstrip to change.
  ~ : PMIOPort  Side=Left
  "~ " : PMIOPort  Port=2  Side=Right
  MGController1 : Outport
  wires:
  PCC Measurements and PCC Breaker/1(" mPCC") -> Microgrid Controller/3("mPCC ")
  Microgrid Controller/2(Vref) -> BESS and Controller/3(Vref)
  [CtrlRoom] -> BESS and Controller/1(CntrlRmIN)
  BESS and Controller/1(mBESS) -> Bus Creator/1, [BESS]  "BESS"
  Bus Creator/1 -> MGController1/1
  [CtrlRoom] -> Bus Selector/1
  Bus Selector/1 -> Simulink-PS Converter/1  "<SubstationBrk>"
  ControlRoom/1 -> [CtrlRoom]
  [CtrlRoom] -> Microgrid Controller/1(CntrlRmIN)
  [BESS] -> Microgrid Controller/2(BESS)
  Microgrid Controller/4(MGCtrl) -> [Controller]  "Controller"
  [Controller] -> Bus Creator/2
  Microgrid Controller/5(BreakerControl) -> [cBreaker]
  [cBreaker] -> PCC Measurements and PCC Breaker/1(cBreaker)
  Microgrid Controller/1(PQref) -> BESS and Controller/2(PQref)
  Microgrid Controller/3(fref) -> BESS and Controller/4(f0)
  connections:
  PCC Measurements and PCC Breaker/RConn1 -- BESS and Controller/LConn1 -- Circuit Breaker (Three-Phase)/LConn2
  Transformer and Disconnectors/RConn1 -- PCC Measurements and PCC Breaker/LConn1
  ~/RConn1 -- Transformer and Disconnectors/LConn1
  Simulink-PS Converter/RConn1 -- Circuit Breaker (Three-Phase)/LConn1
  Circuit Breaker (Three-Phase)/RConn1 -- "~ "/RConn1

== system IndustrialMicrogrid/MG1 Unit Substation ==
  Bus Element In3 : Inport  PortName=ControlRoom  Element=UnitSubstationBrk1
  Bus Element In1 : Inport  PortName=ControlRoom  Element=UnitSubstationBrk2
  Circuit Breaker (Three-Phase) : ee_lib/Switches & Breakers/Circuit Breaker (Three-Phase)  R_closed=0.001 Ohm  G_open=1e-6 1/Ohm  threshold=0.5 V  breaker_behavior=ee.enum.switches.breakerBehavior.zeroCrossingEnable
      settings: InternalSimscapePortConfiguration="{\"Bottom\":[],\"Left\":[{\"id\":\"vT\",\"label\":\"vT\",\"type\":\"input\"},{\"id\":\"N1\",\"label\":\"~1\",\"type\":\"foundation.electrical.three_phase\"}],\"Right\":[{\"id\":\"N2\",\"label\":\"~2\",\"type\":\"foundation.electrical.three_phase\"}],\"Top\":[]}"
  Circuit Breaker (Three-Phase)1 : ee_lib/Switches & Breakers/Circuit Breaker (Three-Phase)  R_closed=0.001 Ohm  G_open=1e-6 1/Ohm  threshold=0.5 V  breaker_behavior=ee.enum.switches.breakerBehavior.zeroCrossingEnable
      settings: InternalSimscapePortConfiguration="{\"Bottom\":[],\"Left\":[{\"id\":\"vT\",\"label\":\"vT\",\"type\":\"input\"},{\"id\":\"N1\",\"label\":\"~1\",\"type\":\"foundation.electrical.three_phase\"}],\"Right\":[{\"id\":\"N2\",\"label\":\"~2\",\"type\":\"foundation.electrical.three_phase\"}],\"Top\":[]}"
  Line X/R=1.44 1 : ee_lib/Passive/RLC Assemblies/RLC (Three-Phase)  component_structure=ee.enum.rlc.structure.SeriesRL  R=microgrid.rLine Ohm  L=microgrid.lLine H  C=1 F  R_parasitic=1e-6 Ohm  G_parasitic=1e-5 1/Ohm  IL_specify=on  IL_priority=High  IL=[0, 0, 0] A  IL_nominal_specify=off  IL_nominal_unit=A  IL_nominal_value=1  VC_specify=on  VC_priority=High  VC=[0, 0, 0] V  VC_nominal_specify=off  VC_nominal_unit=V  VC_nominal_value=1
      settings: InternalSimscapePortConfiguration="{\"Bottom\":[],\"Left\":[{\"id\":\"N1\",\"label\":\"~1\",\"type\":\"foundation.electrical.three_phase\"}],\"Right\":[{\"id\":\"N2\",\"label\":\"~2\",\"type\":\"foundation.electrical.three_phase\"}],\"Top\":[]}"
  Line X/R=1.44 2 : ee_lib/Passive/RLC Assemblies/RLC (Three-Phase)  component_structure=ee.enum.rlc.structure.SeriesRL  R=microgrid.rLine*0.2 Ohm  L=microgrid.lLine*0.2 H  C=1 F  R_parasitic=1e-6 Ohm  G_parasitic=1e-5 1/Ohm  IL_specify=on  IL_priority=High  IL=[0, 0, 0] A  IL_nominal_specify=off  IL_nominal_unit=A  IL_nominal_value=1  VC_specify=on  VC_priority=High  VC=[0, 0, 0] V  VC_nominal_specify=off  VC_nominal_unit=V  VC_nominal_value=1
      settings: InternalSimscapePortConfiguration="{\"Bottom\":[],\"Left\":[{\"id\":\"N1\",\"label\":\"~1\",\"type\":\"foundation.electrical.three_phase\"}],\"Right\":[{\"id\":\"N2\",\"label\":\"~2\",\"type\":\"foundation.electrical.three_phase\"}],\"Top\":[]}"
  Low-Pass Filter (Discrete or Continuous) : eeGeneralControl/Low-Pass Filter (Discrete or Continuous)  K=1  T=0.1  B=inf  A=-inf  init_option=Inherited from block input  x0=0  Ts=Ts
  Low-Pass Filter (Discrete or Continuous)1 : eeGeneralControl/Low-Pass Filter (Discrete or Continuous)  K=1  T=0.1  B=inf  A=-inf  init_option=Inherited from block input  x0=0  Ts=Ts
  PS-Simulink Converter8 : nesl_utility_internal/PS-Simulink Converter  PhysicalDomain=network_engine_domain  SubClassName=ps_output  LeftPortType=input  RightPortType=output  PseudoPeriodic=off  Frequencies=[]  VectorFormat=1-D array  Unit=MW  AffineConversion=off
  PS-Simulink Converter9 : nesl_utility_internal/PS-Simulink Converter  PhysicalDomain=network_engine_domain  SubClassName=ps_output  LeftPortType=input  RightPortType=output  PseudoPeriodic=off  Frequencies=[]  VectorFormat=1-D array  Unit=MV*A  AffineConversion=off
  Power Sensor (Three-Phase)2 : ee_lib/Sensors & Transducers/Power Sensor (Three-Phase)  load_type=ee.enum.passive.type_balanced.balanced  f0=60 Hz  config=ee.enum.with_neutral.no  rho=1
      settings: InternalSimscapePortConfiguration="{\"Bottom\":[],\"Left\":[{\"id\":\"N1\",\"label\":\"~1\",\"type\":\"foundation.electrical.three_phase\"}],\"Right\":[{\"id\":\"N2\",\"label\":\"~2\",\"type\":\"foundation.electrical.three_phase\"}],\"Top\":[{\"id\":\"Pm\",\"label\":\"P\",\"type\":\"output\"},{\"id\":\"Qm\",\"label\":\"Q\",\"type\":\"output\"}]}"
  Simulink-PS Converter : nesl_utility_internal/Simulink-PS Converter  PhysicalDomain=network_engine_domain  SubClassName=ps_input  LeftPortType=input  RightPortType=output  PseudoPeriodic=off  Frequencies=[]  NoiseDistribution=none  NoiseParameters=[]  Unit=1  AffineConversion=off  FilteringAndDerivatives=provide  SimscapeFilterOrder=1  InputFilterTimeConstant=0.001  UdotUserProvided=0
  Simulink-PS Converter1 : nesl_utility_internal/Simulink-PS Converter  PhysicalDomain=network_engine_domain  SubClassName=ps_input  LeftPortType=input  RightPortType=output  PseudoPeriodic=off  Frequencies=[]  NoiseDistribution=none  NoiseParameters=[]  Unit=1  AffineConversion=off  FilteringAndDerivatives=provide  SimscapeFilterOrder=1  InputFilterTimeConstant=0.001  UdotUserProvided=0
  Two-Winding Transformer (Three-Phase)1 : ee_lib/Passive/Transformers/Two-Winding Transformer (Three-Phase)  SRated=microgrid.unitSubstationTransformerRating A*V  FRated=microgrid.frequency Hz  Winding1Connection=ee.enum.windingconnection.Y  VRated1=microgrid.unitSubstationTransformerPrimaryVoltage V  Winding2Connection=ee.enum.windingconnection.Y  VRated2=microgrid.unitSubstationTransformerSecondaryVoltage V  CoreType=ee.enum.coretype.threelimb  pu_Rw1=microgrid.unitSubstationPrimaryResistance  pu_Rw2=microgrid.unitSubstationPrimaryReactance  leakage_reactance_option=ee.enum.transformer_leakage.include  pu_Xl1=microgrid.unitSubstationSecondaryResistance  pu_Xl2=microgrid.unitSubstationSecondaryReactance  magnetizing_resistance_option=ee.enum.transformer_magnetizingResistance.include  pu_Rm=500  magnetizing_reactance_option=ee.enum.transformer_magnetizingReactance.include  saturation_option=ee.enum.transformer_saturation.exclude  pu_Xm=500  current_data=[0, .002, 1, 2]  magnetic_flux_data=[0, 1.2, 1.5, 1.51]  pu_X0=0.5  i1_specify=on  i1_priority=None  i1=[0, 0, 0] A  i1_nominal_specify=off  i1_nominal_unit=A  i1_nominal_value=1  i2_specify=on  i2_priority=None  i2=[0, 0, 0] A  i2_nominal_specify=off  i2_nominal_unit=A  i2_nominal_value=1  phi_specify=off  phi_priority=None  phi=[0, 0, 0]  phi_nominal_specify=off  phi_nominal_unit=1  phi_nominal_value=1  power_dissipated_specify=off  power_dissipated_priority=None  power_dissipated=0 W  power_dissipated_nominal_specify=off  power_dissipated_nominal_unit=W  power_dissipated_nominal_value=1
      settings: InternalSimscapePortConfiguration="{\"Bottom\":[],\"Left\":[{\"id\":\"N1\",\"label\":\"~1\",\"type\":\"foundation.electrical.three_phase\"}],\"Right\":[{\"id\":\"N2\",\"label\":\"~2\",\"type\":\"foundation.electrical.three_phase\"}],\"Top\":[]}"
  "~ " : PMIOPort  Side=Left
  ~ : PMIOPort  Port=2  Side=Right
  " ~ " : PMIOPort  Port=3  Side=Right
  Out Bus Element2 : Outport  PortName=mtieline1  Element=activepower
  Out Bus Element3 : Outport  PortName=mtieline1  Element=reactivepower
  wires:
  Bus Element In3/1 -> Simulink-PS Converter/1
  Bus Element In1/1 -> Simulink-PS Converter1/1
  Low-Pass Filter (Discrete or Continuous)/1 -> Out Bus Element2/1
  PS-Simulink Converter9/1 -> Low-Pass Filter (Discrete or Continuous)1/1
  PS-Simulink Converter8/1 -> Low-Pass Filter (Discrete or Continuous)/1
  Low-Pass Filter (Discrete or Continuous)1/1 -> Out Bus Element3/1
  connections:
  Line X/R=1.44 2/LConn1 -- "~ "/RConn1
  Simulink-PS Converter1/RConn1 -- Circuit Breaker (Three-Phase)1/LConn1
  Circuit Breaker (Three-Phase)/RConn1 -- Line X/R=1.44 1/LConn1
  Simulink-PS Converter/RConn1 -- Circuit Breaker (Three-Phase)/LConn1
  Circuit Breaker (Three-Phase)/LConn2 -- Line X/R=1.44 2/RConn1 -- Circuit Breaker (Three-Phase)1/LConn2
  Circuit Breaker (Three-Phase)1/RConn1 -- Two-Winding Transformer (Three-Phase)1/LConn1
  ~/RConn1 -- Two-Winding Transformer (Three-Phase)1/RConn1
  PS-Simulink Converter8/LConn1 -- Power Sensor (Three-Phase)2/LConn2
  PS-Simulink Converter9/LConn1 -- Power Sensor (Three-Phase)2/LConn3
  Power Sensor (Three-Phase)2/LConn1 -- Line X/R=1.44 1/RConn1
  Power Sensor (Three-Phase)2/RConn1 -- " ~ "/RConn1

== system IndustrialMicrogrid/MG2 Main Grid ==
  Electrical Reference1 : fl_lib/Electrical/Electrical Elements/Electrical Reference
  Main Grid Frequency : Constant  Value=grid.frequency  SampleTime=-1
  Programmable Voltage Source (Three-Phase)2 : ee_lib/Sources/Programmable Voltage Source (Three-Phase)  magnitude_type=ee.enum.timechanging.constant  vline_rms=grid.voltageSource V  magn_ramp=1 V/s  magn_step=1 V  magn_modu_magn=1 V  magn_modu_freq=1 Hz  magn_t1=1 s  magn_t2=2 s  frequency_type=ee.enum.timechanging.external  freq=50 Hz  freq_ramp=1 Hz/s  freq_step=1 Hz  freq_modu_magn=1 Hz  freq_modu_freq=1 Hz  freq_t1=1 s  freq_t2=2 s  phase_type=ee.enum.timechanging.constant  shift=0 deg  phase_ramp=1 deg/s  phase_step=1 deg  phase_modu_magn=1 deg  phase_modu_freq=1 Hz  phase_t1=1 s  phase_t2=2 s  impedance_option=1  SShortCircuit=100e6 A*V  XR=15  R=0.01 Ohm  L=3.97e-4*0.1 H  G_parasitic=1e-6 1/Ohm  harmonic_option=0  harmonic_orders=[5, 7, 11, 13]  harmonic_ratios=[.1, .1, .1, .1]  harmonic_shifts=[0, 0, 0, 0] deg  harmonic_sequences=[1, 1, 1, 1]  harmonic_t1=-inf s  harmonic_t2=inf s  I_specify=on  I_priority=None  I=[0, 0, 0] A  I_nominal_specify=off  I_nominal_unit=A  I_nominal_value=1  V_specify=on  V_priority=None  V=[0, 0, 0] V  V_nominal_specify=off  V_nominal_unit=V  V_nominal_value=1
      settings: InternalSimscapePortConfiguration="{\"Bottom\":[],\"Left\":[{\"id\":\"ext_freq\",\"label\":\"F\",\"type\":\"input\"},{\"id\":\"n\",\"label\":\"n\",\"type\":\"foundation.electrical.electrical\"}],\"Right\":[{\"id\":\"N\",\"label\":\"~\",\"type\":\"foundation.electrical.three_phase\"}],\"Top\":[]}"
  Simulink-PS Converter : nesl_utility_internal/Simulink-PS Converter  PhysicalDomain=network_engine_domain  SubClassName=ps_input  LeftPortType=input  RightPortType=output  PseudoPeriodic=off  Frequencies=[]  NoiseDistribution=none  NoiseParameters=[]  Unit=1  AffineConversion=off  FilteringAndDerivatives=provide  SimscapeFilterOrder=1  InputFilterTimeConstant=0.001  UdotUserProvided=0
  Source impedance and Line X/R=18.8 : ee_lib/Passive/RLC Assemblies/RLC (Three-Phase)  component_structure=ee.enum.rlc.structure.SeriesRL  R=grid.rMV Ohm  L=grid.lMV1 H  C=1e-6 F  R_parasitic=1e-6 Ohm  G_parasitic=1e-6 1/Ohm  IL_specify=on  IL_priority=High  IL=[0, 0, 0] A  IL_nominal_specify=off  IL_nominal_unit=A  IL_nominal_value=1  VC_specify=off  VC_priority=High  VC=[0, 0, 0] V  VC_nominal_specify=off  VC_nominal_unit=V  VC_nominal_value=1
      settings: InternalSimscapePortConfiguration="{\"Bottom\":[],\"Left\":[{\"id\":\"N1\",\"label\":\"~1\",\"type\":\"foundation.electrical.three_phase\"}],\"Right\":[{\"id\":\"N2\",\"label\":\"~2\",\"type\":\"foundation.electrical.three_phase\"}],\"Top\":[]}"
  ref : PMIOPort  Side=Left
  ~ : PMIOPort  Port=2  Side=Right
  wires:
  Main Grid Frequency/1 -> Simulink-PS Converter/1
  connections:
  ref/RConn1 -- Electrical Reference1/LConn1 -- Programmable Voltage Source (Three-Phase)2/LConn2
  Source impedance and Line X/R=18.8/LConn1 -- Programmable Voltage Source (Three-Phase)2/RConn1
  Source impedance and Line X/R=18.8/RConn1 -- ~/RConn1
  Simulink-PS Converter/RConn1 -- Programmable Voltage Source (Three-Phase)2/LConn1
